simulink model "ejemplodiscreto"  (R2016a)
settings: Solver=ode45  StartTime=0.0  StopTime=10  RelTol=1e-3
values from neighbouring files (symbols this model uses):
  a = [-1 0;0 2]    [ejemplodiscretro.m]
  b = [1;1]    [ejemplodiscretro.m]
  c = [1,1]    [ejemplodiscretro.m]
  ki = kt(:,3:3)    [ejemplodiscretro.m]
  kidis = ktdis(:,3:3)    [ejemplodiscretro.m]
  kp = kt(:,1:2)    [ejemplodiscretro.m]
  kpdis = ktdis(:,1:2)    [ejemplodiscretro.m]
  tm = 0.1    [ejemplodiscretro.m]
undefined symbols (not defined in the file or in its folder): adis, bdis, cdis
settings Model: Creator=Dell  LastModifiedBy=jtombe
settings DataIOCC: LimitDataPoints=on  SaveFormat=Array  SignalLoggingSaveFormat=ModelDataLogs
settings OptimizationCC: ExpressionDepthLimit=2147483647
settings DebuggingCC: UnderspecifiedInitializationDetection=Classic  MergeDetectMultiDrivingBlocksExec=none  SolverPrmCheckMsg=warning  FcnCallInpInsideContextMsg=UseLocalSettings  StateNameClashWarn=warning
settings HardwareCC: ProdBitPerPointer=32  ProdLargestAtomicFloat=None  ProdIntDivRoundTo=Undefined  ProdEndianess=Unspecified  ProdWordSize=32  ProdHWDeviceType=32-bit Generic
settings ModelReferenceCC: PropagateSignalLabelsOutOfModel=off
settings GRTTargetCC: CombineOutputUpdateFcns=off  GRTInterface=on
settings ConfigComp: CovModelRefEnable=Off  CovSFcnEnable=off

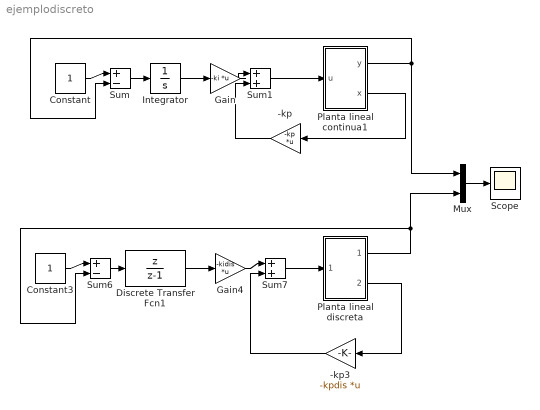
== system ejemplodiscreto ==
  -kp : Gain  Gain=-kp  Multiplication=Matrix(K*u) (u vector)
  -kp3 : Gain  Gain=-kpdis  Multiplication=Matrix(K*u) (u vector)  SampleTime=tm
  Constant : Constant
  Constant3 : Constant  SampleTime=tm
  Discrete Transfer Fcn1 : DiscreteTransferFcn  Numerator=[1 0]  Denominator=[1 -1]  SampleTime=tm
  Gain : Gain  Gain=-ki  Multiplication=Matrix(K*u) (u vector)
  Gain4 : Gain  Gain=-kidis  Multiplication=Matrix(K*u) (u vector)  SampleTime=tm
  Integrator : Integrator
  Mux : Mux  Inputs=2
  Planta lineal continua1 : Subsystem
  Planta lineal discreta : Subsystem
  Scope : Scope
  Sum : Sum  Inputs=|+-
  Sum1 : Sum  Inputs=|++
  Sum6 : Sum  Inputs=|+-
  Sum7 : Sum  Inputs=|++
  wires:
  Constant/1 -> Sum/1
  Sum/1 -> Integrator/1
  Integrator/1 -> Gain/1
  Gain/1 -> Sum1/1
  Sum1/1 -> Planta lineal continua1/1(u)
  -kp/1 -> Sum1/2
  Planta lineal continua1/2(x) -> -kp/1
  Planta lineal continua1/1(y) -> Sum/2, Mux/1
  Constant3/1 -> Sum6/1
  Sum6/1 -> Discrete Transfer Fcn1/1
  Discrete Transfer Fcn1/1 -> Gain4/1
  Gain4/1 -> Sum7/1
  Sum7/1 -> Planta lineal discreta/1(In1)
  -kp3/1 -> Sum7/2
  Planta lineal discreta/1(ydis) -> Mux/2, Sum6/2
  Planta lineal discreta/2(xdis) -> -kp3/1
  Mux/1 -> Scope/1

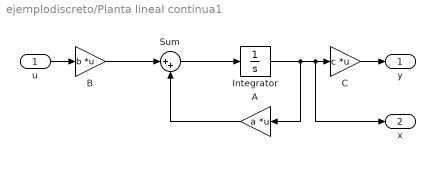
== system ejemplodiscreto/Planta lineal continua1 ==
  u : Inport
  A : Gain  Gain=a  Multiplication=Matrix(K*u) (u vector)
  B : Gain  Gain=b  Multiplication=Matrix(K*u) (u vector)
  C : Gain  Gain=c  Multiplication=Matrix(K*u) (u vector)
  Integrator : Integrator
  Sum : Sum  Inputs=|++
  y : Outport
  x : Outport  Port=2
  wires:
  B/1 -> Sum/1
  Sum/1 -> Integrator/1
  A/1 -> Sum/2
  Integrator/1 -> A/1, C/1, x/1
  u/1 -> B/1
  C/1 -> y/1

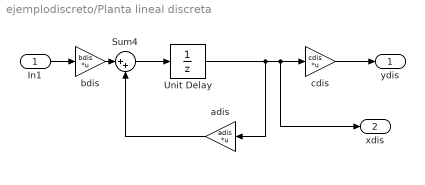
== system ejemplodiscreto/Planta lineal discreta ==
  In1 : Inport
  Sum4 : Sum  Inputs=|++
  Unit Delay : UnitDelay  SampleTime=tm
  adis : Gain  Gain=adis  Multiplication=Matrix(K*u) (u vector)  SampleTime=tm
  bdis : Gain  Gain=bdis  Multiplication=Matrix(K*u) (u vector)  SampleTime=tm
  cdis : Gain  Gain=cdis  Multiplication=Matrix(K*u) (u vector)  SampleTime=tm
  ydis : Outport
  xdis : Outport  Port=2
  wires:
  cdis/1 -> ydis/1
  In1/1 -> bdis/1
  adis/1 -> Sum4/2
  Unit Delay/1 -> cdis/1, xdis/1, adis/1
  Sum4/1 -> Unit Delay/1
  bdis/1 -> Sum4/1
